simulink model "enabledSineDemo"  (R2016b)
settings: Solver=ode5  StartTime=0.0  StopTime=inf  FixedStep=0.001  RelTol=1e-3  EnableMultiTasking=on
libraries: simulink x1, dcpctrl x1
settings Model: SimulationMode=external  Creator=julianleland  LastModifiedBy=julianleland
settings OptimizationCC: LifeSpan=inf
settings DebuggingCC: SFUnexpectedBacktrackingDiag=warning  SFNoUnconditionalDefaultTransitionDiag=warning  SFExecutionAtInitializationDiag=none
settings HardwareCC: ProdBitPerLong=64  ProdHWDeviceType=Intel->x86-64 (Mac OS X)  TargetBitPerLong=64  TargetBitPerPointer=64  TargetIntDivRoundTo=Zero  TargetEndianess=LittleEndian  TargetWordSize=64  TargetHWDeviceType=Intel->x86-64
settings RTWCC: SystemTargetFile=sldrt.tlc  TemplateMakefile=sldrt.tmf  Description=Simulink Desktop Real-Time  RTWCompilerOptimization=on
settings CodeAppCC: MaxIdLength=95
settings SimulinkDesktopRealTimeCC: TargetPreCompLibLocation=/Applications/MATLAB_R2016b.app/toolbox/sldrt/lib/maci64  TargetLangStandard=C89/C90 (ANSI)  SupportVariableSizeSignals=off
settings ConfigComp: CovMetricSettings=dw  CovHtmlReporting=on  CovSaveCumulativeToWorkspaceVar=on  CovSaveSingleToWorkspaceVar=on  CovExternalEMLEnable=off

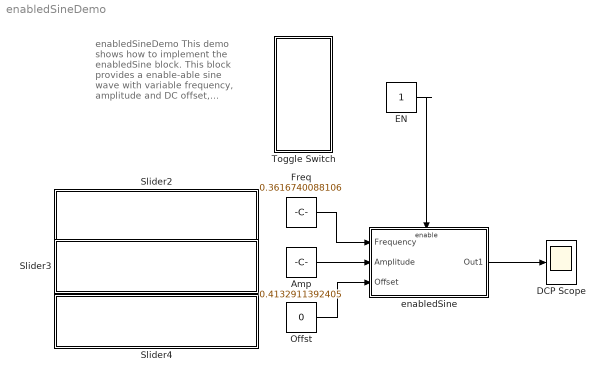
== system enabledSineDemo ==
  note: enabledSineDemo
      | This demo shows how to implement the enabledSine block. This block provides a enable-able sine wave with variable frequency, amplitude and DC offset, which is useful for testing. Enabling resets the wave state to zero.
  Amp : Constant  Value=0.4132911392405
  DCP Scope : Scope
  EN : Constant
  Freq : Constant  Value=0.3616740088106
  Offst : Constant  Value=0
  Slider2 : Subsystem  DialogController=hmiCreateDDGDialog  IsWebBlock=on  mask(MWDashboardBlock){webBlockId=bd791960-66e3-42ca-a5e7-affb25679ee0, webBlockType=slider, ShowInLibBrowser=on, ShowInitialText=on, HMISrcModelName=enabledSineDemo}
      mask prompts: webBlockId "WebBlock Id"; webBlockType "WebBlock Type"; HMISrcModelName "Source Model"
      mask Help: helpview([docroot '/mapfiles/simulink.map'], 'hmi_slider')
      mask Display:
      | if strcmp(get_param(bdroot(gcb),'BlockDiagramType'), 'library')
      |     image([(matlabroot) '/toolbox/simulink/hmi/icons/Slider.png']);
      | end
  Slider3 : Subsystem  DialogController=hmiCreateDDGDialog  IsWebBlock=on  mask(MWDashboardBlock){webBlockId=dbe37d33-4096-4c50-a0e6-912eb045fc7f, webBlockType=slider, ShowInLibBrowser=on, ShowInitialText=on, HMISrcModelName=enabledSineDemo}
      mask prompts: webBlockId "WebBlock Id"; webBlockType "WebBlock Type"; HMISrcModelName "Source Model"
      mask Help: helpview([docroot '/mapfiles/simulink.map'], 'hmi_slider')
      mask Display:
      | if strcmp(get_param(bdroot(gcb),'BlockDiagramType'), 'library')
      |     image([(matlabroot) '/toolbox/simulink/hmi/icons/Slider.png']);
      | end
  Slider4 : Subsystem  DialogController=hmiCreateDDGDialog  IsWebBlock=on  mask(MWDashboardBlock){webBlockId=1c1362f3-7e0f-4c04-8074-7765d65329f4, webBlockType=slider, ShowInLibBrowser=on, ShowInitialText=on, HMISrcModelName=enabledSineDemo}
      mask prompts: webBlockId "WebBlock Id"; webBlockType "WebBlock Type"; HMISrcModelName "Source Model"
      mask Help: helpview([docroot '/mapfiles/simulink.map'], 'hmi_slider')
      mask Display:
      | if strcmp(get_param(bdroot(gcb),'BlockDiagramType'), 'library')
      |     image([(matlabroot) '/toolbox/simulink/hmi/icons/Slider.png']);
      | end
  Toggle Switch : Subsystem  DialogController=hmiCreateDDGDialog  IsWebBlock=on  mask(MWDashboardBlock){webBlockId=ede58e36-eb20-490a-8fe3-ac65bc340523, webBlockType=toggleswitch, ShowInLibBrowser=on, ShowInitialText=on, HMISrcModelName=enabledSineDemo}
      mask prompts: webBlockId "WebBlock Id"; webBlockType "WebBlock Type"; HMISrcModelName "Source Model"
      mask help: SimulinkHMI:dialogs:SwitchDialogDesc
      mask Help: helpview([docroot '/mapfiles/simulink.map'], 'hmi_toggle_switch')
      mask Display:
      | if strcmp(get_param(bdroot(gcb),'BlockDiagramType'), 'library')
      |     image([(matlabroot) '/toolbox/simulink/hmi/icons/ToggleSwitch.png']);
      | end
  enabledSine : Subsystem
  wires:
  enabledSine/1(Out1) -> DCP Scope/1
  EN/1 -> enabledSine/Enable
  Freq/1 -> enabledSine/1(Frequency)
  Amp/1 -> enabledSine/2(Amplitude)
  Offst/1 -> enabledSine/3(Offset)

== system enabledSineDemo/Slider2 ==

== system enabledSineDemo/Slider3 ==

== system enabledSineDemo/Slider4 ==

== system enabledSineDemo/Toggle Switch ==

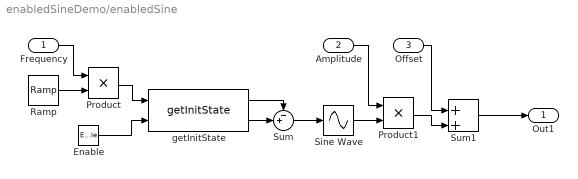
== system enabledSineDemo/enabledSine ==
  Frequency : Inport
  Amplitude : Inport  Port=2
  Offset : Inport  Port=3
  Enable : EnablePort  StatesWhenEnabling=reset  ShowOutputPort=on
  Product : Product
  Product1 : Product
  Ramp : simulink/Sources/Ramp  slope=1  start=0  X0=0
  Sine Wave : Sin  TimeSource=Use external signal  SampleTime=0
  Sum : Sum  Inputs=-+|
  Sum1 : Sum  Inputs=+|+
  getInitState : dcpctrl/getInitState
  Out1 : Outport
  wires:
  Enable/1 -> getInitState/2
  Ramp/1 -> Product/2
  getInitState/2 -> Sum/2
  getInitState/1 -> Sum/1
  Sum/1 -> Sine Wave/1
  Product/1 -> getInitState/1
  Frequency/1 -> Product/1
  Sine Wave/1 -> Product1/2
  Product1/1 -> Sum1/2
  Amplitude/1 -> Product1/1
  Offset/1 -> Sum1/1
  Sum1/1 -> Out1/1
